simulink model "WORKINGSL"  (R2023b)
settings: Solver=VariableStepAuto  StartTime=0.0  StopTime=1900.0  RelTol=1e-3
undefined symbols (not defined in the file): A, Breal, C, K_feedbackOnly, Ki, Kx, L, N_bar, sys
settings Model: Creator=jeppe  LastModifiedBy=jeppe
settings SolverCC: AutoInsertRateTranBlk=on

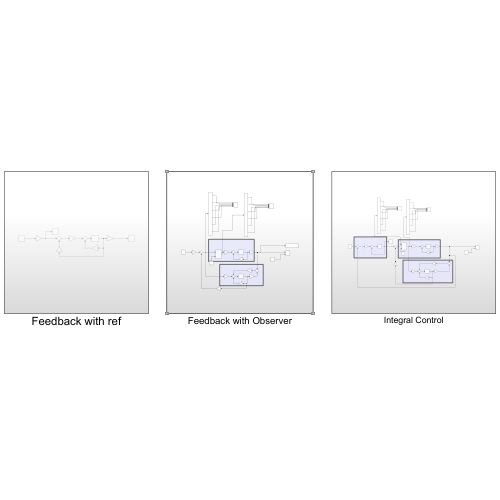
[thumbnail: Simulink's stored preview of the top-level diagram]
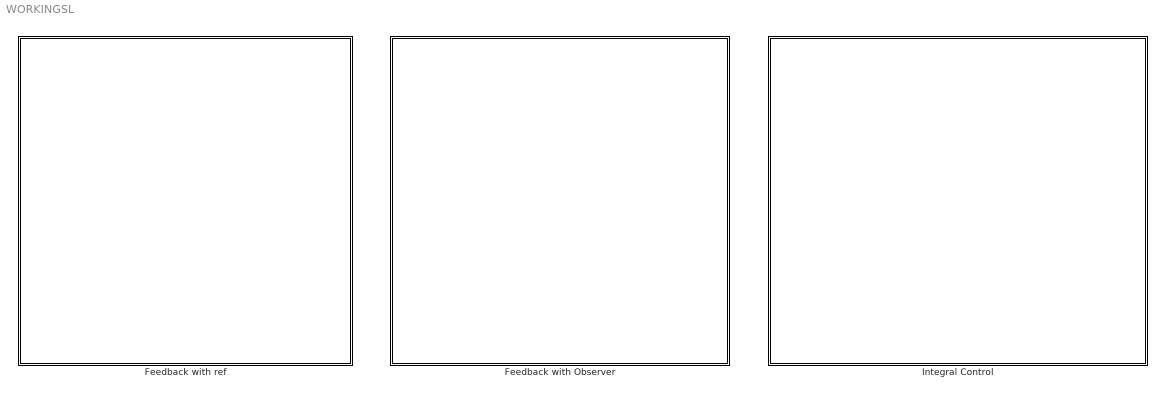
== system WORKINGSL ==
  Feedback with Observer : Subsystem
  Feedback with ref : Subsystem
  Integral Control : Subsystem

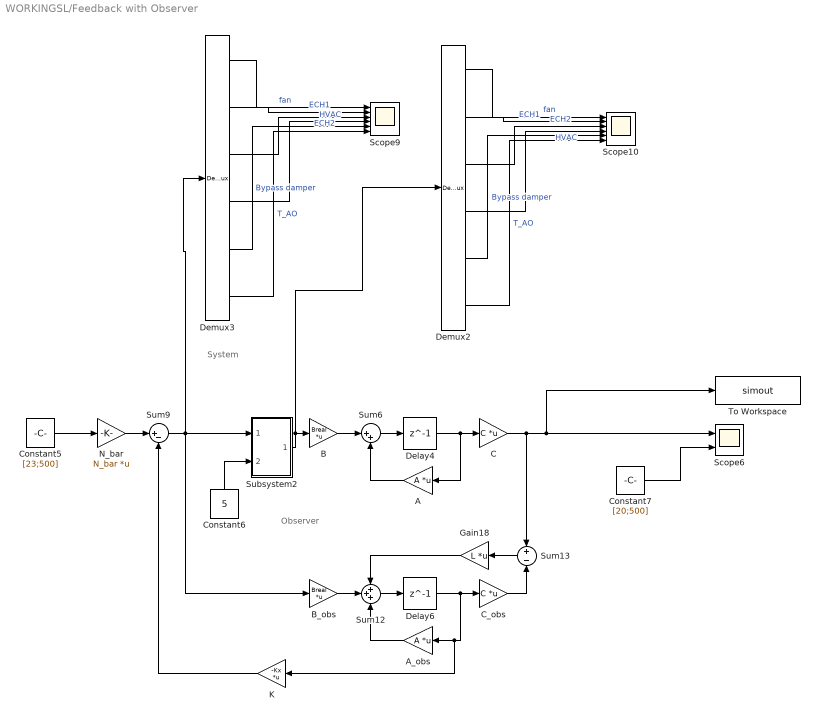
== system WORKINGSL/Feedback with Observer ==
  note: System
  note: Observer
  A : Gain  Gain=A  Multiplication=Matrix(K*u)
  A_obs : Gain  Gain=A  Multiplication=Matrix(K*u)
  B : Gain  Gain=Breal  Multiplication=Matrix(K*u)
  B_obs : Gain  Gain=Breal  Multiplication=Matrix(K*u)
  C : Gain  Gain=C  Multiplication=Matrix(K*u)
  C_obs : Gain  Gain=C  Multiplication=Matrix(K*u)
  Constant5 : Constant  Value=[23;500]
  Constant6 : Constant  Value=5
  Constant7 : Constant  Value=[20;500]
  Delay4 : Delay  DelayLength=1  InitialCondition=C^-1*[18;1000]
  Delay6 : Delay  DelayLength=1  InitialCondition=C^-1*[18;1000]
  Demux2 : Demux  Outputs=6
  Demux3 : Demux  Outputs=6
  Gain18 : Gain  Gain=L  Multiplication=Matrix(K*u)
  K : Gain  Gain=-Kx  Multiplication=Matrix(K*u)
  N_bar : Gain  Gain=N_bar  Multiplication=Matrix(K*u)
  Scope10 : Scope  NumInputPorts=6
  Scope6 : Scope  NumInputPorts=2
  Scope9 : Scope  NumInputPorts=6
  Subsystem2 : Subsystem  TreatAsAtomicUnit=on  ScheduleAs=Periodic partition  PartitionName=Subsystem  SystemSampleTime=15
  Sum12 : Sum  Inputs=+++
  Sum13 : Sum  Inputs=+|-
  Sum6 : Sum  Inputs=|++
  Sum9 : Sum  Inputs=|+-
  To Workspace : ToWorkspace  VariableName=simout  SampleTime=-1
  wires:
  Delay4/1 -> A/1, C/1
  Demux3/6 -> Scope9/6  "T_AO"
  C/1 -> To Workspace/1, Scope6/1, Sum13/1
  Constant6/1 -> Subsystem2/2(T_AO)
  Demux3/2 -> Scope9/2  "ECH1"
  Demux2/6 -> Scope10/6  "T_AO"
  Demux2/3 -> Scope10/3  "ECH2"
  Demux2/4 -> Scope10/4  "HVAC"
  Demux3/3 -> Scope9/3  "ECH2"
  K/1 -> Sum9/2
  Demux2/1 -> Scope10/1  "fan"
  Demux2/5 -> Scope10/5  "Bypass damper"
  Demux3/5 -> Scope9/5  "Bypass damper"
  B/1 -> Sum6/1
  B_obs/1 -> Sum12/2
  Sum9/1 -> Subsystem2/1(signals), Demux3/1, B_obs/1
  Demux3/1 -> Scope9/1  "fan"
  Gain18/1 -> Sum12/1
  Delay6/1 -> A_obs/1, K/1, C_obs/1
  Constant7/1 -> Scope6/2
  Sum6/1 -> Delay4/1
  Sum13/1 -> Gain18/1
  Demux2/2 -> Scope10/2  "ECH1"
  Sum12/1 -> Delay6/1
  A_obs/1 -> Sum12/3
  A/1 -> Sum6/2
  C_obs/1 -> Sum13/2
  Demux3/4 -> Scope9/4  "HVAC"
  Subsystem2/1(Out1) -> Demux2/1, B/1
  Constant5/1 -> N_bar/1
  N_bar/1 -> Sum9/1

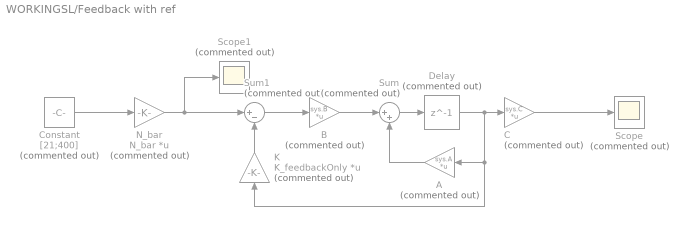
== system WORKINGSL/Feedback with ref ==
  A : Gain  Commented=on  Gain=sys.A  Multiplication=Matrix(K*u)
  B : Gain  Commented=on  Gain=sys.B  Multiplication=Matrix(K*u)
  C : Gain  Commented=on  Gain=sys.C  Multiplication=Matrix(K*u)
  Constant : Constant  Commented=on  Value=[21;400]
  Delay : Delay  Commented=on  DelayLength=1  InitialCondition=0
  K : Gain  Commented=on  Gain=K_feedbackOnly  Multiplication=Matrix(K*u)
  N_bar : Gain  Commented=on  Gain=N_bar  Multiplication=Matrix(K*u)
  Scope : Scope  Commented=on
  Scope1 : Scope  Commented=on
  Sum : Sum  Commented=on  Inputs=|++
  Sum1 : Sum  Commented=on  Inputs=|+-
  wires:
  Delay/1 -> A/1, K/1, C/1
  B/1 -> Sum/1
  N_bar/1 -> Scope1/1, Sum1/1
  C/1 -> Scope/1
  A/1 -> Sum/2
  Constant/1 -> N_bar/1
  Sum1/1 -> B/1
  Sum/1 -> Delay/1
  K/1 -> Sum1/2

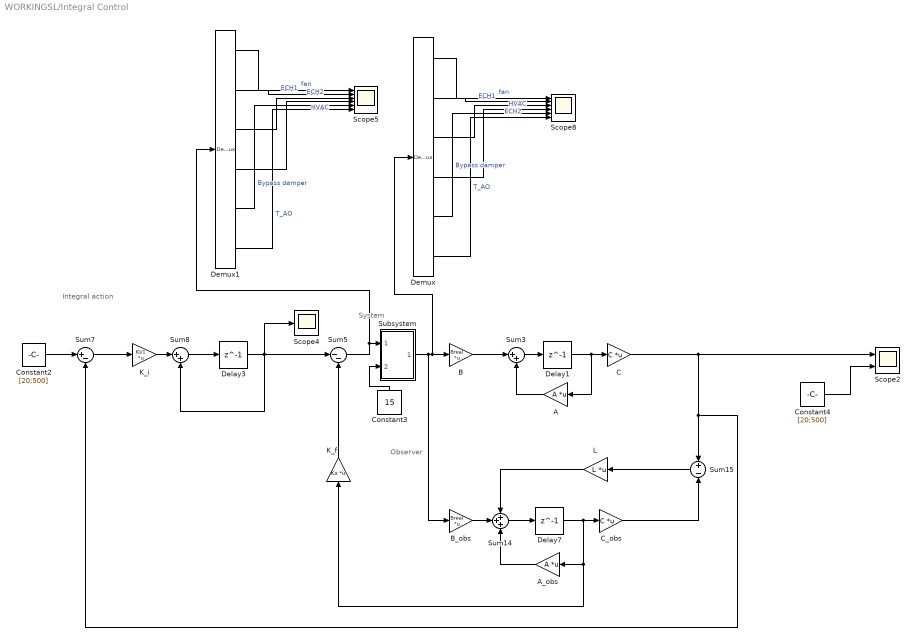
== system WORKINGSL/Integral Control ==
  note: Integral action
  note: System
  note: Observer
  A : Gain  Gain=A  Multiplication=Matrix(K*u)
  A_obs : Gain  Gain=A  Multiplication=Matrix(K*u)
  B : Gain  Gain=Breal  Multiplication=Matrix(K*u)
  B_obs : Gain  Gain=Breal  Multiplication=Matrix(K*u)
  C : Gain  Gain=C  Multiplication=Matrix(K*u)
  C_obs : Gain  Gain=C  Multiplication=Matrix(K*u)
  Constant2 : Constant  Value=[20;500]
  Constant3 : Constant  Value=15
  Constant4 : Constant  Value=[20;500]
  Delay1 : Delay  DelayLength=1  InitialCondition=C^-1*[18;1000]
  Delay3 : Delay  DelayLength=1  InitialCondition=0
  Delay7 : Delay  DelayLength=1  InitialCondition=C^-1*[18;1000]
  Demux : Demux  Outputs=6
  Demux1 : Demux  Outputs=6
  K_f : Gain  Gain=Kx  Multiplication=Matrix(K*u)
  K_i : Gain  Gain=Ki/1  Multiplication=Matrix(K*u)
  L : Gain  Gain=L  Multiplication=Matrix(K*u)
  Scope2 : Scope  NumInputPorts=2
  Scope4 : Scope
  Scope5 : Scope  NumInputPorts=6
  Scope8 : Scope  NumInputPorts=6
  Subsystem : Subsystem  TreatAsAtomicUnit=on  ScheduleAs=Periodic partition  PartitionName=Subsystem  SystemSampleTime=15
  Sum14 : Sum  Inputs=+++
  Sum15 : Sum  Inputs=+|-
  Sum3 : Sum  Inputs=|++
  Sum5 : Sum  Inputs=|--
  Sum7 : Sum  Inputs=|+-
  Sum8 : Sum  Inputs=|++
  wires:
  Sum5/1 -> Demux1/1, Subsystem/1(signals)
  Demux/4 -> Scope8/4  "HVAC"
  K_i/1 -> Sum8/1
  Subsystem/1(Out1) -> B_obs/1, Demux/1, B/1
  Delay3/1 -> Sum8/2, Sum5/1, Scope4/1
  Demux/1 -> Scope8/1  "fan"
  Delay7/1 -> A_obs/1, K_f/1, C_obs/1
  C/1 -> Scope2/1, Sum15/1, Sum7/2
  Sum3/1 -> Delay1/1
  A_obs/1 -> Sum14/3
  Demux/6 -> Scope8/6  "T_AO"
  B/1 -> Sum3/1
  Demux1/1 -> Scope5/1  "fan"
  Sum7/1 -> K_i/1
  Demux1/2 -> Scope5/2  "ECH1"
  Demux/2 -> Scope8/2  "ECH1"
  Demux1/5 -> Scope5/5  "Bypass damper"
  Constant4/1 -> Scope2/2
  Demux1/3 -> Scope5/3  "ECH2"
  Demux/3 -> Scope8/3  "ECH2"
  Demux1/6 -> Scope5/6  "T_AO"
  Demux1/4 -> Scope5/4  "HVAC"
  L/1 -> Sum14/1
  Constant3/1 -> Subsystem/2(T_AO)
  Sum14/1 -> Delay7/1
  Delay1/1 -> A/1, C/1
  Constant2/1 -> Sum7/1
  Sum8/1 -> Delay3/1
  K_f/1 -> Sum5/2
  C_obs/1 -> Sum15/2
  B_obs/1 -> Sum14/2
  Demux/5 -> Scope8/5  "Bypass damper"
  A/1 -> Sum3/2
  Sum15/1 -> L/1

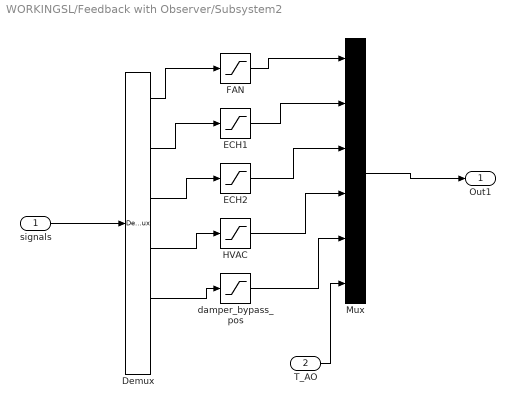
== system WORKINGSL/Feedback with Observer/Subsystem2 ==
  signals : Inport
  T_AO : Inport  Port=2
  Demux : Demux  Outputs=6
  ECH1 : Saturate  UpperLimit=100  LowerLimit=0
  ECH2 : Saturate  UpperLimit=100  LowerLimit=0
  FAN : Saturate  UpperLimit=100  LowerLimit=30
  HVAC : Saturate  UpperLimit=100  LowerLimit=-100
  Mux : Mux  Inputs=6
  damper_bypass_pos : Saturate  UpperLimit=100  LowerLimit=0
  Out1 : Outport
  wires:
  signals/1 -> Demux/1
  Demux/1 -> FAN/1
  Demux/2 -> ECH1/1
  Demux/3 -> ECH2/1
  Demux/4 -> HVAC/1
  Demux/5 -> damper_bypass_pos/1
  FAN/1 -> Mux/1
  ECH1/1 -> Mux/2
  ECH2/1 -> Mux/3
  HVAC/1 -> Mux/4
  damper_bypass_pos/1 -> Mux/5
  T_AO/1 -> Mux/6
  Mux/1 -> Out1/1

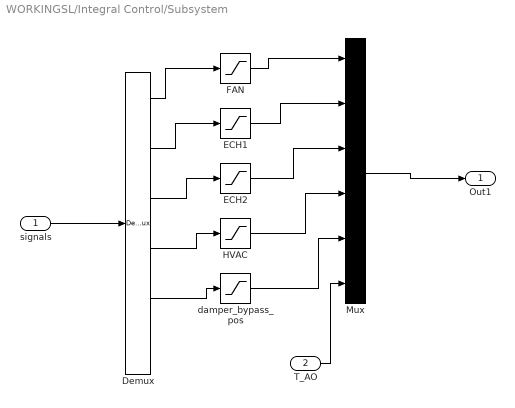
== system WORKINGSL/Integral Control/Subsystem ==
  signals : Inport
  T_AO : Inport  Port=2
  Demux : Demux  Outputs=6
  ECH1 : Saturate  UpperLimit=100  LowerLimit=0
  ECH2 : Saturate  UpperLimit=100  LowerLimit=0
  FAN : Saturate  UpperLimit=100  LowerLimit=30
  HVAC : Saturate  UpperLimit=100  LowerLimit=-100
  Mux : Mux  Inputs=6
  damper_bypass_pos : Saturate  UpperLimit=100  LowerLimit=0
  Out1 : Outport
  wires:
  signals/1 -> Demux/1
  Demux/1 -> FAN/1
  Demux/2 -> ECH1/1
  Demux/3 -> ECH2/1
  Demux/4 -> HVAC/1
  Demux/5 -> damper_bypass_pos/1
  FAN/1 -> Mux/1
  ECH1/1 -> Mux/2
  ECH2/1 -> Mux/3
  HVAC/1 -> Mux/4
  damper_bypass_pos/1 -> Mux/5
  T_AO/1 -> Mux/6
  Mux/1 -> Out1/1
